simulink model "psk"  (R2018a)
settings: Solver=FixedStepDiscrete  StartTime=0.0  StopTime=10.0  RelTol=1e-3
libraries: commchan3 x1, simulink x1, dspfdesign x1, commseqgen3 x1
settings Model: Creator=Владимир  LastModifiedBy=Владимир

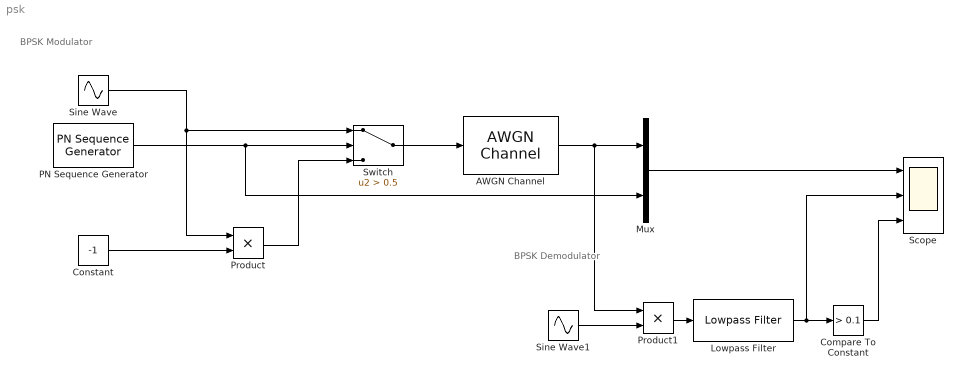
== system psk ==
  note: BPSK Demodulator
  note: BPSK Modulator
  AWGN Channel : commchan3/AWGN Channel  InputProcessing=Columns as channels (frame based)  seed=67  noiseMode="Signal to noise ratio  (Eb/No)"  EbNodB=40  EsNodB=10  SNRdB=10  bitsPerSym=1  Ps=1  Tsym=1  variance=1
  Compare To Constant : simulink/Logic and Bit Operations/Compare To Constant  relop=>  const=0.1  OutDataTypeStr=boolean
  Constant : Constant  Value=-1
  Lowpass Filter : dspfdesign/Lowpass Filter  FilterType=FIR  DesignForMinimumOrder=on  FilterOrder=50  PassbandFrequency=2  StopbandFrequency=5  PassbandRipple=1  StopbandAttenuation=60  InheritSampleRate=on  SampleRate=1000  SimulateUsing=Interpreted execution  roundingMode=Floor  coeffsDataTypeStr=fixdt(1,16)
  Mux : Mux  Inputs=2
  PN Sequence Generator : commseqgen3/PN Sequence Generator  poly='z^6 + z + 1'  ini_sta=[0 0 0 0 0 1]  outBitMaskSource=Dialog parameter  shift=0  outVarSiz=off  maxOutSizeMode=Dialog parameter  maxOutSize=[10 1]  Ts=0.5  sampPerFrame=1  reset=off  bitPackedOutputs=off  outDataType=double  numPackedBits=8  bitPackDataSigned=off  bitPackedOutDType=double
      settings: SourceProductName=Communications System Toolbox
  Product : Product
  Product1 : Product
  Scope : Scope  NumInputPorts=3
  Sine Wave : Sin  Frequency=2*pi*2  SampleTime=0.001
  Sine Wave1 : Sin  Frequency=2*pi*2  SampleTime=0.001
  Switch : Switch  Criteria=u2 > Threshold  Threshold=0.5
  wires:
  Sine Wave/1 -> Switch/1, Product/1
  PN Sequence Generator/1 -> Mux/2, Switch/2
  Constant/1 -> Product/2
  Product/1 -> Switch/3
  Mux/1 -> Scope/1
  Switch/1 -> AWGN Channel/1
  AWGN Channel/1 -> Mux/1, Product1/1
  Sine Wave1/1 -> Product1/2
  Product1/1 -> Lowpass Filter/1
  Compare To Constant/1 -> Scope/3
  Lowpass Filter/1 -> Compare To Constant/1, Scope/2
